simulink library "drd"  (Simulink 8.1)
settings: Solver=ode1  StartTime=0.0  StopTime=Inf  FixedStep=0.001  RelTol=1e-3
PostLoadFcn:
  | , if any(exist('dsrtsu_mdlpostloadfcn', 'file') == [2, 3, 6]), try dsrtsu_mdlpostloadfcn('Execute', bdroot); catch fprintf('Error in PostLoadFcn (dsrtsu_mdlpostloadfcn) for model "%s":\n %s\n', bdroot, lasterr); end, end,
undefined symbols (not defined in the file or in its folder): KACC_ACCCriticalClearance_m, ZERO_FLOAT
libraries: ins x1, icd x1, its x1, nif x1
settings Model: DSRTSU_INTERNAL_RTI_VER=450  DSRTSU_INTERNAL_RTI_TYPE=rti1401  Creator=AT015555  LastModifiedBy=AT015555

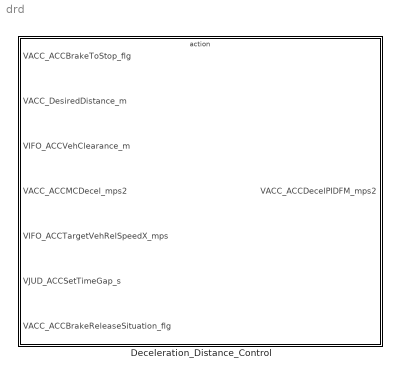
== system drd ==
  Deceleration_Distance_Control : Subsystem  TreatAsAtomicUnit=on

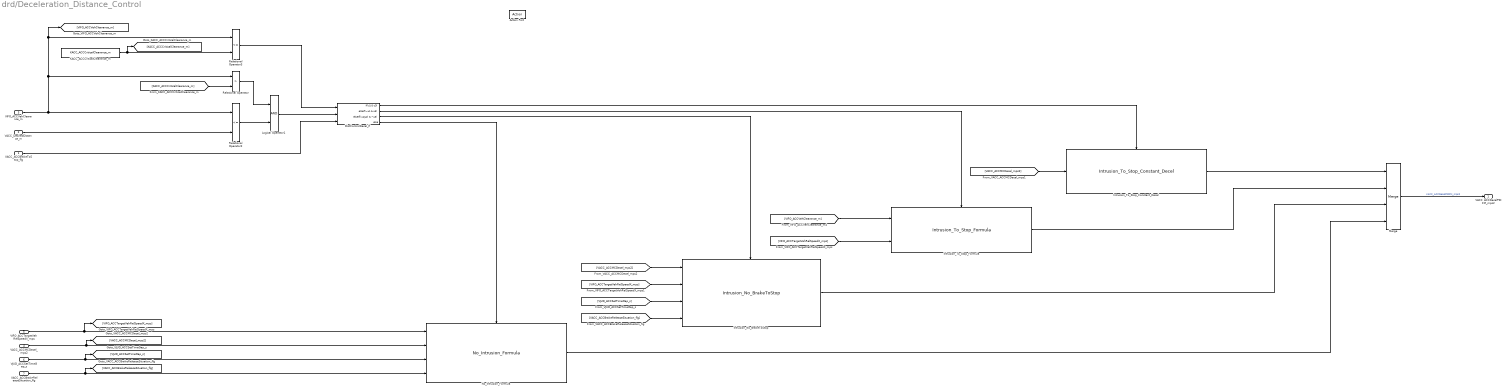
== system drd/Deceleration_Distance_Control ==
  VACC_ACCBrakeToStop_flg : Inport
  VACC_DesiredDistance_m : Inport  Port=2
  VIFO_ACCVehClearance_m : Inport  Port=3
  VACC_ACCMCDecel_mps2 : Inport  Port=4
  VIFO_ACCTargetVehRelSpeedX_mps : Inport  Port=5
  VJUD_ACCSetTimeGap_s : Inport  Port=6
  VACC_ACCBrakeReleaseSituation_flg : Inport  Port=7
  Action Port : ActionPort
  DistControlDecel_If : If  NumInputs=3  IfExpression=u1 & u3  ElseIfExpressions=~u1 & u3,(u1|u2) & ~u3
  Intrusion_No_BrakeToStop : ins/Intrusion_No_BrakeToStop
  Intrusion_To_Stop_Constant_Decel : icd/Intrusion_To_Stop_Constant_Decel
  Intrusion_To_Stop_Formula : its/Intrusion_To_Stop_Formula
  KACC_ACCCriticalClearance_m : Constant  Value=KACC_ACCCriticalClearance_m
  Logical Operator1 : Logic  AllPortsSameDT=off  OutDataTypeStr=boolean
  Merge : Merge  Inputs=4
  No_Intrusion_Formula : nif/No_Intrusion_Formula
  Relational Operator : RelationalOperator  Operator=>  OutDataTypeStr=boolean
  Relational Operator2 : RelationalOperator  Operator=<=  OutDataTypeStr=boolean
  Relational Operator3 : RelationalOperator  Operator=<=  OutDataTypeStr=boolean
  VACC_ACCDecelPIDFM_mps2 : Outport  OutputWhenDisabled=reset  InitialOutput=ZERO_FLOAT
  wires:
  VIFO_ACCVehClearance_m/1 -> [VIFO_ACCVehClearance_m], Relational Operator3/1, Relational Operator/1, Relational Operator2/1
  VACC_DesiredDistance_m/1 -> Relational Operator2/2
  Relational Operator2/1 -> Logical Operator1/2
  VACC_ACCBrakeToStop_flg/1 -> DistControlDecel_If/3
  Relational Operator/1 -> Logical Operator1/1
  Logical Operator1/1 -> DistControlDecel_If/2
  VACC_ACCMCDecel_mps2/1 -> No_Intrusion_Formula/2, [VACC_ACCMCDecel_mps2]
  VIFO_ACCTargetVehRelSpeedX_mps/1 -> No_Intrusion_Formula/1, [VIFO_ACCTargetVehRelSpeedX_mps]
  DistControlDecel_If/4 -> No_Intrusion_Formula/Action
  DistControlDecel_If/3 -> Intrusion_No_BrakeToStop/Action
  DistControlDecel_If/2 -> Intrusion_To_Stop_Formula/Action
  [VACC_ACCMCDecel_mps2] -> Intrusion_No_BrakeToStop/1
  [VIFO_ACCTargetVehRelSpeedX_mps] -> Intrusion_To_Stop_Formula/2
  [VIFO_ACCVehClearance_m] -> Intrusion_To_Stop_Formula/1
  DistControlDecel_If/1 -> Intrusion_To_Stop_Constant_Decel/Action
  No_Intrusion_Formula/1 -> Merge/4
  Intrusion_No_BrakeToStop/1 -> Merge/3
  Intrusion_To_Stop_Formula/1 -> Merge/2
  Intrusion_To_Stop_Constant_Decel/1 -> Merge/1
  Merge/1 -> VACC_ACCDecelPIDFM_mps2/1  "VACC_ACCDecelPIDFM_mps2"
  Relational Operator3/1 -> DistControlDecel_If/1
  [VIFO_ACCTargetVehRelSpeedX_mps] -> Intrusion_No_BrakeToStop/2
  KACC_ACCCriticalClearance_m/1 -> Relational Operator3/2, [KACC_ACCCriticalClearance_m]
  [KACC_ACCCriticalClearance_m] -> Relational Operator/2
  VJUD_ACCSetTimeGap_s/1 -> No_Intrusion_Formula/3, [VJUD_ACCSetTimeGap_s]
  [VJUD_ACCSetTimeGap_s] -> Intrusion_No_BrakeToStop/3
  [VACC_ACCMCDecel_mps2] -> Intrusion_To_Stop_Constant_Decel/1
  VACC_ACCBrakeReleaseSituation_flg/1 -> No_Intrusion_Formula/4, [VACC_ACCBrakeReleaseSituation_flg]
  [VACC_ACCBrakeReleaseSituation_flg] -> Intrusion_No_BrakeToStop/4
